simulink model "HydICengine"  (R2023b)
settings: Solver=ode3  StartTime=0.0  StopTime=1*sim_time  FixedStep=(120/engine_speed)/2000  RelTol=1e-3  EnableMultiTasking=on
values from neighbouring files (symbols this model uses):
  engine_speed = 1500    [RunModel.m]
  sim_time = stepsize * (2*1000 - 1)    (= 0.07996)    [RunModel.m]
settings Model: Creator=htsauto  LastModifiedBy=sami
settings SolverCC: AlgebraicLoopSolver=TrustRegion
settings DataIOCC: LimitDataPoints=on  SaveFormat=Array  SignalLoggingSaveFormat=ModelDataLogs  ReturnWorkspaceOutputs=off
settings OptimizationCC: ExpressionDepthLimit=2147483647  LifeSpan=inf
settings DebuggingCC: UnderspecifiedInitializationDetection=Classic  MergeDetectMultiDrivingBlocksExec=none  SolverPrmCheckMsg=warning  FcnCallInpInsideContextMsg=warning  UnconnectedInputMsg=warning  UnconnectedOutputMsg=warning  UnconnectedLineMsg=warning  StateNameClashWarn=warning  SFUnexpectedBacktrackingDiag=warning  SFNoUnconditionalDefaultTransitionDiag=warning  ArithmeticOperatorsInVariantConditions=warning
settings HardwareCC: ProdBitPerPointer=32  ProdBitPerSizeT=32  ProdBitPerPtrDiffT=32  ProdLargestAtomicFloat=None  ProdIntDivRoundTo=Undefined  ProdEndianess=Unspecified  ProdWordSize=32  ProdHWDeviceType=32-bit Generic
settings ModelReferenceCC: EnableRefExpFcnMdlSchedulingChecks=on  PropagateSignalLabelsOutOfModel=off
settings SFSimCC: SimUseLocalCustomCode=off  CustomCodeUndefinedFunction=UseInterfaceOnly
settings RTWCC: RTWUseLocalCustomCode=off
settings CodeAppCC: StateflowObjectComments=on
settings GRTTargetCC: TargetLangStandard=C89/C90 (ANSI)  CombineOutputUpdateFcns=off  GRTInterface=on
settings ConfigComp: CovMetricSettings=dw  CovSaveCumulativeToWorkspaceVar=on  CovSaveSingleToWorkspaceVar=on  CovExternalEMLEnable=off  CovSFcnEnable=off

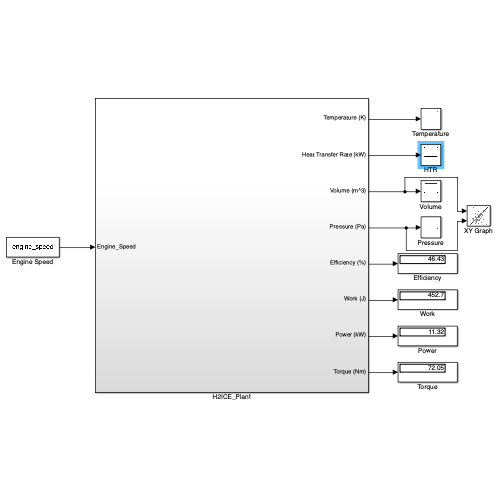
[thumbnail: Simulink's stored preview of the top-level diagram]
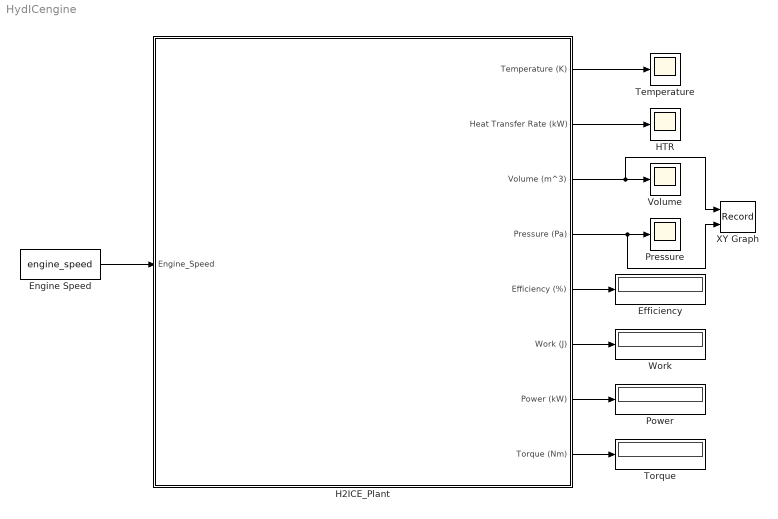
== system HydICengine ==
  Efficiency : Display
  Engine Speed : Constant  Value=engine_speed
  H2ICE_Plant : Subsystem
  HTR : Scope
  Power : Display
  Pressure : Scope
  Temperature : Scope
  Torque : Display
  Volume : Scope
  Work : Display
  XY Graph : Record  FileSettingsInternal="{\"entries\":[{\"content\":{\"excelSettings\":{\"content\":{},\"type\":\"Streamout.ExcelSettings\"}},\"type\":\"Streamout.FileSettingStorage\",\"uuid\":\"\"}],\"packageUris\":[\"http:\\/\\/schema.mathworks.com\\/mf0\\/streamout_blocks\\/R2020a\"],\"version\":\"1.0\"}"  Layout=[1 1]  SignalsInternal="{\"entries\":[{\"content\":{\"signals\":[{\"content\":{\"blockPath\":[],\"dimensions\":[1],\"domain\":\"\",\"lineColor\":\"#fe330a\",\"plots\":[ 1 ],\"port\":1,\"sid\":[\"\"],\"signalID\":1,\"signalName\":\"H2ICE_Plant:3\"},\"type\":\"RecordBlkView.Signal\",\"uuid\":\"\"},{\"content\":{\"blockPath\":[],\"dimensions\":[1],\"domain\":\"\",\"lineColor\":\"#fe330a\",\"plots\":[ 1 ],\"port\":2,\"sid\":[\"\"],\"signalID\":2,\"signalName\":\"H2ICE_Plant:4\"},\"type\":\"RecordBlkView.Signal\",\"uuid\":\"\"}]},\"type\":\"RecordBlkView.InputSignals\",\"uuid\":\"\"}],\"packageUris\":[\"http:\\/\\/schema.mathworks.com\\/mf0\\/streamout_blocks\\/R2020a\"],\"version\":\"1.0\"}"  VisualizationBindings="{\"xyplotplugin\":{\"info\":[{\"series\":[{\"bindingParametersList\":[{\"parameter\":\"X-Axis\",\"signalID\":1,\"signalName\":\"H2ICE_Plant:3\"},{\"parameter\":\"Y-Axis\",\"signalID\":2,\"signalName\":\"H2ICE_Plant:4\"}],\"seriesID\":0}],\"subplotID\":1}]}}"  CompatibilityTag=XY
  wires:
  H2ICE_Plant/8(Torque (Nm)) -> Torque/1
  H2ICE_Plant/7(Power (kW)) -> Power/1
  H2ICE_Plant/6(Work (J)) -> Work/1
  H2ICE_Plant/5(Efficiency (%)) -> Efficiency/1
  H2ICE_Plant/3(Volume (m^3)) -> Volume/1, XY Graph/1
  H2ICE_Plant/4(Pressure (Pa)) -> Pressure/1, XY Graph/2
  H2ICE_Plant/1(Temperature (K)) -> Temperature/1
  Engine Speed/1 -> H2ICE_Plant/1(Engine_Speed)
  H2ICE_Plant/2(Heat Transfer Rate (kW)) -> HTR/1

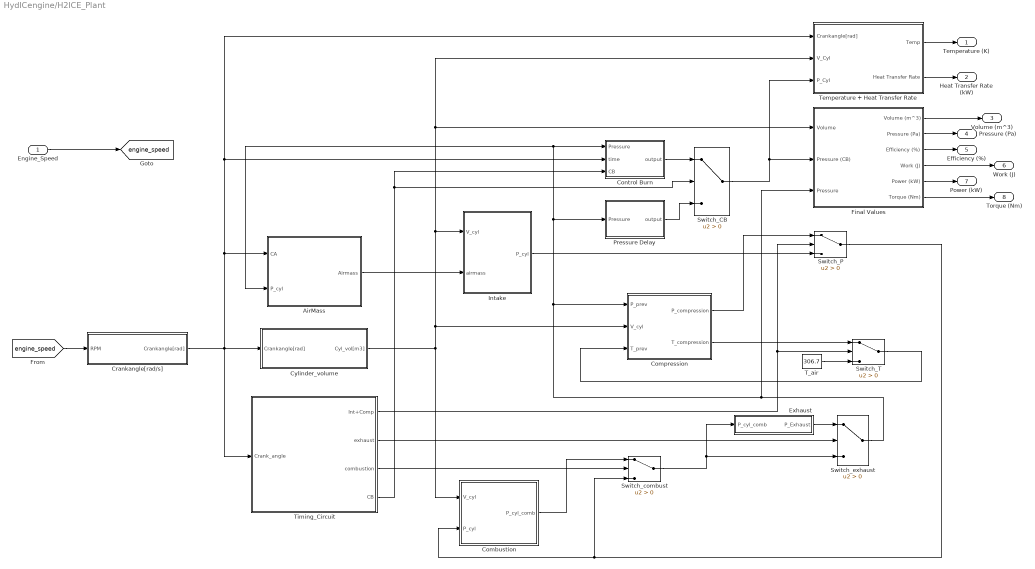
== system HydICengine/H2ICE_Plant ==
  Engine_Speed : Inport
  AirMass : Subsystem
  Combustion : Subsystem
  Compression : Subsystem
  Control Burn : Subsystem
  Crankangle[rad/s] : Subsystem
  Cylinder_volume : Subsystem
  Exhaust : Subsystem
  Final Values : Subsystem
  Intake : Subsystem
  Pressure Delay : Subsystem
  Switch_CB : Switch  Criteria=u2 > Threshold  SaturateOnIntegerOverflow=off  InputSameDT=off
  Switch_P : Switch  Criteria=u2 > Threshold  SaturateOnIntegerOverflow=off  InputSameDT=off
  Switch_T : Switch  Criteria=u2 > Threshold  SaturateOnIntegerOverflow=off  InputSameDT=off
  Switch_combust : Switch  Criteria=u2 > Threshold  SaturateOnIntegerOverflow=off  InputSameDT=off
  Switch_exhaust : Switch  Criteria=u2 > Threshold  SaturateOnIntegerOverflow=off  InputSameDT=off
  T_air : Constant  Value=306.7
  Temperature + Heat Transfer Rate : Subsystem
  Timing_Circuit : Subsystem
  Temperature (K) : Outport
  Heat Transfer Rate (kW) : Outport  Port=2
  Volume (m^3) : Outport  Port=3
  Pressure (Pa) : Outport  Port=4
  Efficiency (%) : Outport  Port=5
  Work (J) : Outport  Port=6
  Power (kW) : Outport  Port=7
  Torque (Nm) : Outport  Port=8
  tag scope: engine_speed=global
  wires:
  [engine_speed] -> Crankangle[rad/s]/1(RPM)
  Switch_exhaust/1 -> Final Values/3(Pressure), AirMass/2(P_cyl), Control Burn/1(Pressure), Pressure Delay/1(Pressure), Compression/1(P_prev)
  Combustion/1(P_cyl_comb) -> Switch_combust/1
  Switch_T/1 -> Compression/3(T_prev)
  Switch_combust/1 -> Exhaust/1(P_cyl_comb), Switch_exhaust/3
  Compression/2(T_compression) -> Switch_T/1
  AirMass/1(Airmass) -> Intake/2(airmass)
  Cylinder_volume/1(Cyl_vol[m3]) -> Compression/2(V_cyl), Temperature + Heat Transfer Rate/2(V_Cyl), Final Values/1(Volume), Intake/1(V_cyl), Combustion/1(V_cyl)
  Exhaust/1(P_Exhaust) -> Switch_exhaust/1
  Compression/1(P_compression) -> Switch_P/1
  Crankangle[rad/s]/1(Crankangle[rad]) -> Timing_Circuit/1(Crank_angle), Temperature + Heat Transfer Rate/1(Crankangle[rad]), Control Burn/2(time), AirMass/1(CA), Cylinder_volume/1(Crankangle[rad])
  T_air/1 -> Switch_T/3
  Intake/1(P_cyl) -> Switch_P/3
  Timing_Circuit/3(combustion) -> Switch_combust/2
  Switch_P/1 -> Combustion/2(P_cyl), Switch_combust/3
  Timing_Circuit/2(exhaust) -> Switch_exhaust/2
  Timing_Circuit/1(Int+Comp) -> Switch_P/2, Switch_T/2
  Temperature + Heat Transfer Rate/2(Heat Transfer Rate) -> Heat Transfer Rate (kW)/1
  Temperature + Heat Transfer Rate/1(Temp) -> Temperature (K)/1
  Final Values/2(Pressure (Pa)) -> Pressure (Pa)/1
  Final Values/1(Volume (m^3)) -> Volume (m^3)/1
  Engine_Speed/1 -> [engine_speed]
  Final Values/3(Efficiency (%)) -> Efficiency (%)/1
  Final Values/4(Work (J)) -> Work (J)/1
  Final Values/5(Power (kW)) -> Power (kW)/1
  Final Values/6(Torque (Nm)) -> Torque (Nm)/1
  Switch_CB/1 -> Temperature + Heat Transfer Rate/3(P_Cyl), Final Values/2(Pressure (CB))
  Timing_Circuit/4(CB) -> Control Burn/3(CB), Switch_CB/2
  Control Burn/1(output) -> Switch_CB/1
  Pressure Delay/1(output) -> Switch_CB/3

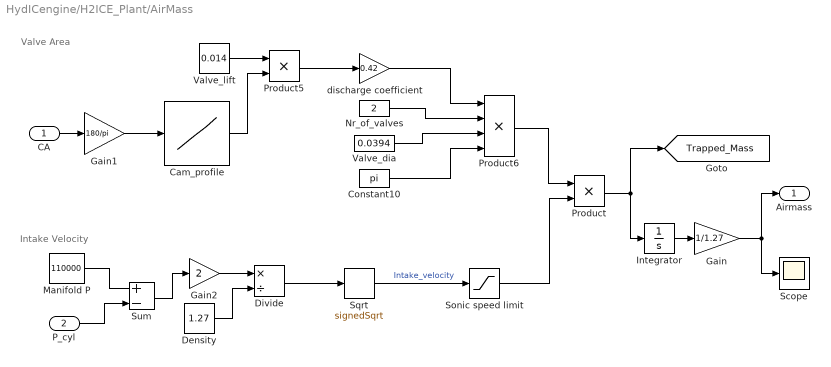
== system HydICengine/H2ICE_Plant/AirMass ==
  note: Intake Velocity
  note: Valve Area
  CA : Inport
  P_cyl : Inport  Port=2
  Cam_profile : Lookup_n-D  NumberOfTableDimensions=1  BreakpointsForDimension1=[0,10,20,30,40,50,60,70,80,90,100,110,120,130,140,150,160,170,180,190,200,210]  Table=[0,0.05,0.1,0.2,0.3,0.5,0.65,0.8,0.9,0.95,1,1,1,1,0.9,0.8,0.65,0.5,0.3,0.2,0.1,0]  ExtrapMethod=Clip  UseLastTableValue=on  RndMeth=Simplest
  Constant10 : Constant  Value=pi
  Density : Constant  Value=1.27
  Divide : Product  Inputs=*/
  Gain : Gain  Gain=1/1.27
  Gain1 : Gain  Gain=180/pi
  Gain2 : Gain  Gain=2
  Integrator : Integrator
  Manifold P : Constant  Value=110000
  Nr_of_valves : Constant  Value=2
  Product : Product
  Product5 : Product  RndMeth=Zero
  Product6 : Product  Inputs=4  RndMeth=Zero
  Scope : Scope
  Sonic speed limit : Saturate  UpperLimit=343.439  LowerLimit=-343.439
  Sqrt : Sqrt  Operator=signedSqrt
  Sum : Sum  Inputs=+-
  Valve_dia : Constant  Value=0.0394
  Valve_lift : Constant  Value=0.014
  discharge coefficient : Gain  Gain=0.42
  Airmass : Outport
  tag scope: Trapped_Mass=global
  wires:
  Gain/1 -> Scope/1, Airmass/1
  Product/1 -> [Trapped_Mass], Integrator/1
  Constant10/1 -> Product6/4
  Valve_dia/1 -> Product6/3
  Nr_of_valves/1 -> Product6/2
  discharge coefficient/1 -> Product6/1
  Sonic speed limit/1 -> Product/2
  Divide/1 -> Sqrt/1
  Sqrt/1 -> Sonic speed limit/1  "Intake_velocity"
  Product5/1 -> discharge coefficient/1
  Cam_profile/1 -> Product5/2
  Product6/1 -> Product/1
  Gain2/1 -> Divide/1
  Valve_lift/1 -> Product5/1
  Gain1/1 -> Cam_profile/1
  Sum/1 -> Gain2/1
  Density/1 -> Divide/2
  Integrator/1 -> Gain/1
  CA/1 -> Gain1/1
  P_cyl/1 -> Sum/2
  Manifold P/1 -> Sum/1

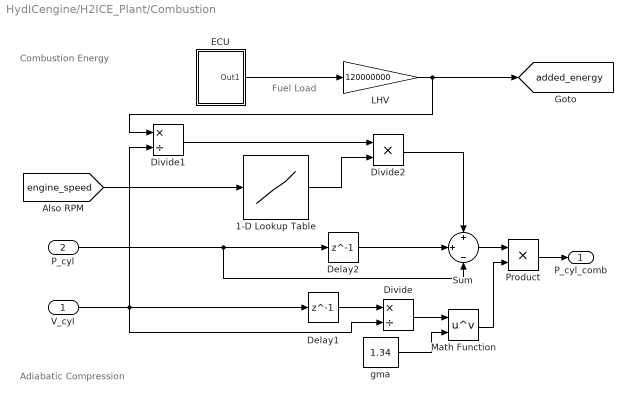
== system HydICengine/H2ICE_Plant/Combustion ==
  note: Combustion Energy
  note: Fuel Load
  note: Adiabatic Compression
  V_cyl : Inport
  P_cyl : Inport  Port=2
  1-D Lookup Table : Lookup_n-D  NumberOfTableDimensions=1  BreakpointsForDimension1=[1000, 1500, 1801, 2000, 2500, 3000, 3500, 4000, 4500, 5000]  Table=[0.36, 0.28, 0.25, 0.23, 0.21, 0.19, 0.19, 0.19, 0.19, 0.19]  InternalRulePriority=Speed  RndMeth=Simplest
  Delay1 : Delay  DelayLength=1
  Delay2 : Delay  DelayLength=1
  Divide : Product  Inputs=*/
  Divide1 : Product  Inputs=*/
  Divide2 : Product  Inputs=**
  ECU : Subsystem
      mask Display: image('Screenshot 2025-03-29 at 14.23.46.png');
  LHV : Gain  Gain=120000000
  Math Function : Math  Operator=pow  SignedPower=on
  Product : Product
  Sum : Sum  Inputs=+|+|-
  gma : Constant  Value=1.34
  P_cyl_comb : Outport
  tag scope: added_energy=global
  wires:
  Delay1/1 -> Divide/1
  Divide/1 -> Math Function/1
  Product/1 -> P_cyl_comb/1
  V_cyl/1 -> Delay1/1, Divide/2, Divide1/2
  Sum/1 -> Product/1
  Delay2/1 -> Sum/2
  Math Function/1 -> Product/2
  gma/1 -> Math Function/2
  P_cyl/1 -> Delay2/1, Sum/3
  [engine_speed] -> 1-D Lookup Table/1
  Divide1/1 -> Divide2/1
  Divide2/1 -> Sum/1
  1-D Lookup Table/1 -> Divide2/2
  LHV/1 -> [added_energy], Divide1/1
  ECU/1(Out1) -> LHV/1

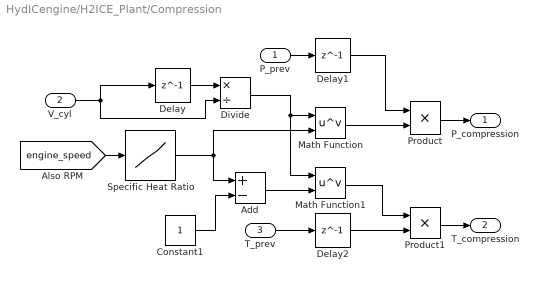
== system HydICengine/H2ICE_Plant/Compression ==
  P_prev : Inport
  V_cyl : Inport  Port=2
  T_prev : Inport  Port=3
  Add : Sum  Inputs=+-
  Constant1 : Constant
  Delay : Delay  DelayLength=1  InitialCondition=0
  Delay1 : Delay  DelayLength=1  InitialCondition=0
  Delay2 : Delay  DelayLength=1
  Divide : Product  Inputs=*/
  Math Function : Math  Operator=pow  SignedPower=on
  Math Function1 : Math  Operator=pow  SignedPower=on
  Product : Product
  Product1 : Product
  Specific Heat Ratio : Lookup_n-D  NumberOfTableDimensions=1  BreakpointsForDimension1=[1000, 1500, 1801, 2000, 2500, 3000, 3500, 4000, 4500, 5000]  Table=[1.6, 1.53, 1.47, 1.45, 1.41, 1.39, 1.38, 1.38, 1.38, 1.38]  InternalRulePriority=Speed  RndMeth=Simplest
  P_compression : Outport
  T_compression : Outport  Port=2
  wires:
  Product1/1 -> T_compression/1
  Delay2/1 -> Product1/2
  Delay1/1 -> Product/1
  Add/1 -> Math Function1/2
  Product/1 -> P_compression/1
  Divide/1 -> Math Function/1, Math Function1/1
  P_prev/1 -> Delay1/1
  Constant1/1 -> Add/2
  V_cyl/1 -> Delay/1, Divide/2
  Math Function/1 -> Product/2
  Math Function1/1 -> Product1/1
  Specific Heat Ratio/1 -> Math Function/2, Add/1
  Delay/1 -> Divide/1
  [engine_speed] -> Specific Heat Ratio/1
  T_prev/1 -> Delay2/1

== system HydICengine/H2ICE_Plant/Control Burn ==
  Pressure : Inport
  time : Inport  Port=2
  CB : Inport  Port=3
  Constant : Constant  Value=6.317760114
  Constant1 : Constant  Value=6.311473785
  Display : Display
  Display1 : Display
  MATLAB Function : MATLAB Function  TreatAsAtomicUnit=on
  MATLAB Function1 : MATLAB Function  TreatAsAtomicUnit=on
  MATLAB Function2 : MATLAB Function  TreatAsAtomicUnit=on
  Scope1 : Scope
  Scope3 : Scope
  output : Outport
  wires:
  Pressure/1 -> MATLAB Function/2(input), MATLAB Function2/1(input)
  Constant/1 -> MATLAB Function/1(targetTime)
  time/1 -> MATLAB Function/3(time), MATLAB Function2/2(time)
  Constant1/1 -> MATLAB Function2/3(targetTime)
  MATLAB Function2/1(output) -> MATLAB Function1/3(minPressure), Display1/1
  MATLAB Function2/2(trigger) -> Scope3/1
  MATLAB Function/1(output) -> MATLAB Function1/1(maxPressure), Display/1
  MATLAB Function1/1(output) -> output/1
  CB/1 -> MATLAB Function1/2(rangeActive)
  MATLAB Function/2(trigger) -> Scope1/1

== system HydICengine/H2ICE_Plant/Crankangle[rad//s] ==
  RPM : Inport
  Clock : Clock
  Display : Display
  Product : Product
  RPM to rad : Gain  Gain=(2*pi/60)
  Scope : Scope
  Crankangle[rad] : Outport
  wires:
  RPM/1 -> RPM to rad/1
  RPM to rad/1 -> Product/1
  Clock/1 -> Product/2
  Product/1 -> Display/1, Scope/1, Crankangle[rad]/1

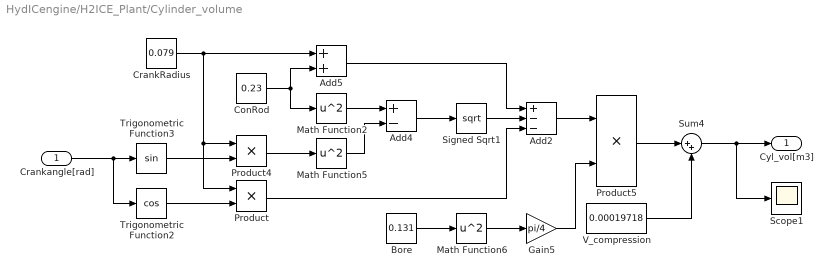
== system HydICengine/H2ICE_Plant/Cylinder_volume ==
  Crankangle[rad] : Inport
  Add2 : Sum  Inputs=+--
  Add4 : Sum  Inputs=+-
  Add5 : Sum
  Bore : Constant  Value=0.131
  ConRod : Constant  Value=0.23
  CrankRadius : Constant  Value=0.079
  Gain5 : Gain  Gain=pi/4
  Math Function2 : Math  Operator=square  SignedPower=on
  Math Function5 : Math  Operator=square  SignedPower=on
  Math Function6 : Math  Operator=square  SignedPower=on
  Product : Product
  Product4 : Product
  Product5 : Product
  Scope1 : Scope
  Signed Sqrt1 : Sqrt
  Sum4 : Sum  Inputs=|++
  Trigonometric Function2 : Trigonometry  Operator=cos
  Trigonometric Function3 : Trigonometry
  V_compression : Constant  Value=0.00019718
  Cyl_vol[m3] : Outport
  wires:
  Product5/1 -> Sum4/1
  Sum4/1 -> Scope1/1, Cyl_vol[m3]/1
  Gain5/1 -> Product5/2
  Add2/1 -> Product5/1
  Math Function6/1 -> Gain5/1
  ConRod/1 -> Add5/2, Math Function2/1
  Add4/1 -> Signed Sqrt1/1
  Product4/1 -> Math Function5/1
  Math Function2/1 -> Add4/1
  V_compression/1 -> Sum4/2
  Add5/1 -> Add2/1
  Product/1 -> Add2/3
  Signed Sqrt1/1 -> Add2/2
  Math Function5/1 -> Add4/2
  Trigonometric Function2/1 -> Product/2
  Crankangle[rad]/1 -> Trigonometric Function2/1, Trigonometric Function3/1
  CrankRadius/1 -> Add5/1, Product4/1, Product/1
  Bore/1 -> Math Function6/1
  Trigonometric Function3/1 -> Product4/2

== system HydICengine/H2ICE_Plant/Exhaust ==
  P_cyl_comb : Inport
  Clock : Clock
  Constant : Constant  Value=sim_time
  Gain : Gain  Gain=0.74
  Relational Operator : RelationalOperator  OutDataTypeStr=boolean  RndMeth=Simplest  InputSameDT=off
  Triggered Subsystem : Subsystem  TreatAsAtomicUnit=on
  P_Exhaust : Outport
  wires:
  Constant/1 -> Gain/1
  Clock/1 -> Relational Operator/1
  Gain/1 -> Relational Operator/2
  Relational Operator/1 -> Triggered Subsystem/Trigger
  P_cyl_comb/1 -> Triggered Subsystem/1(In1)
  Triggered Subsystem/1(Out1) -> P_Exhaust/1

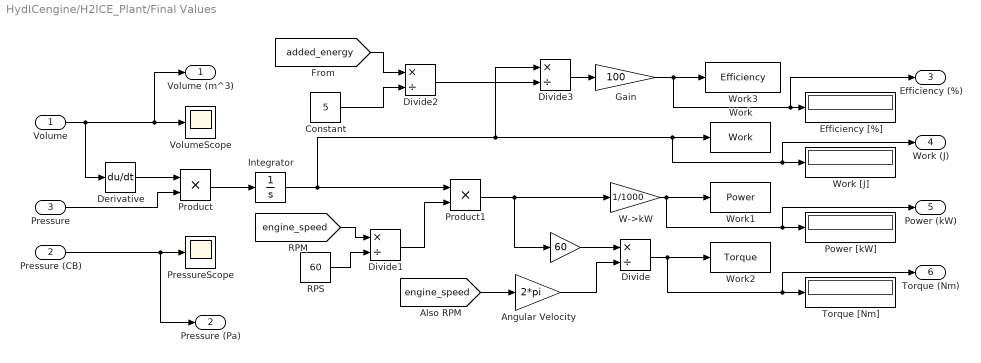
== system HydICengine/H2ICE_Plant/Final Values ==
  Volume : Inport
  Pressure (CB) : Inport  Port=2
  Pressure : Inport  Port=3
  "      " : Gain  Gain=60
  "      W->kW" : Gain  Gain=1/1000
  Angular Velocity : Gain  Gain=2*pi
  Constant : Constant  Value=5
  Derivative : Derivative
  Divide{,1..3} (4 alike) : Product  Inputs=*/
  Efficiency [%] : Display
  Gain : Gain  Gain=100
  Integrator : Integrator
  Power [kW] : Display
  PressureScope : Scope
  Product : Product
  Product1 : Product
  RPS : Constant  Value=60
  Torque [Nm] : Display
  VolumeScope : Scope
  Work : ToWorkspace  VariableName=Work  SampleTime=-1
      settings: MaxDataPoints=1
  "Work [J] " : Display
  Work1 : ToWorkspace  VariableName=Power  SampleTime=-1
      settings: MaxDataPoints=1
  Work2 : ToWorkspace  VariableName=Torque  SampleTime=-1
      settings: MaxDataPoints=1
  Work3 : ToWorkspace  VariableName=Efficiency  SampleTime=-1
      settings: MaxDataPoints=1
  Volume (m^3) : Outport
  Pressure (Pa) : Outport  Port=2
  Efficiency (%) : Outport  Port=3
  Work (J) : Outport  Port=4
  Power (kW) : Outport  Port=5
  Torque (Nm) : Outport  Port=6
  wires:
  Integrator/1 -> Work/1, Work (J)/1, "Work [J] "/1, Divide3/1, Product1/1
  Volume/1 -> Derivative/1, Volume (m^3)/1, VolumeScope/1
  Derivative/1 -> Product/1
  Product/1 -> Integrator/1
  "      "/1 -> Divide/1
  [engine_speed] -> Angular Velocity/1
  Angular Velocity/1 -> Divide/2
  [engine_speed] -> Divide1/1
  RPS/1 -> Divide1/2
  Divide1/1 -> Product1/2
  "      W->kW"/1 -> Power (kW)/1, Power [kW]/1, Work1/1
  [added_energy] -> Divide2/1
  Constant/1 -> Divide2/2
  Divide2/1 -> Divide3/2
  Divide3/1 -> Gain/1
  Gain/1 -> Work3/1, Efficiency (%)/1, Efficiency [%]/1
  Pressure (CB)/1 -> Pressure (Pa)/1, PressureScope/1
  Divide/1 -> Work2/1, Torque (Nm)/1, Torque [Nm]/1
  Pressure/1 -> Product/2
  Product1/1 -> "      W->kW"/1, "      "/1

== system HydICengine/H2ICE_Plant/Intake ==
  note: pre-combustion cylinder pressure
  V_cyl : Inport
  airmass : Inport  Port=2
  Display : Display
  Product7 : Product  Inputs=/***  RndMeth=Zero
  R : Constant  Value=287
  Scope : Scope
  Sum6 : Sum  Inputs=|++
  T_air : Constant  Value=306.7
  To Workspace : ToWorkspace  VariableName=AirMass  SampleTime=-1
      settings: MaxDataPoints=1
  m_0 : Constant  Value=0.00022401
  P_cyl : Outport
  wires:
  R/1 -> Product7/3
  T_air/1 -> Product7/4
  Product7/1 -> Display/1, P_cyl/1, Scope/1
  Sum6/1 -> Product7/2
  m_0/1 -> Sum6/1
  airmass/1 -> To Workspace/1, Sum6/2
  V_cyl/1 -> Product7/1

== system HydICengine/H2ICE_Plant/Pressure Delay ==
  Pressure : Inport
  Delay : Delay  DelayLength=24  InitialCondition=0
  Switch : Switch  Criteria=u2 > Threshold  SaturateOnIntegerOverflow=off  InputSameDT=off
  output : Outport
  wires:
  Pressure/1 -> Delay/1, Switch/1
  Delay/1 -> Switch/3
  [CB2] -> Switch/2
  Switch/1 -> output/1

== system HydICengine/H2ICE_Plant/Temperature + Heat Transfer Rate ==
  Crankangle[rad] : Inport
  V_Cyl : Inport  Port=2
  P_Cyl : Inport  Port=3
  Heat Transfer Rate Subsystem : Subsystem
  Heat_Transfer_Rate : Scope
  Temp Subsystem : Subsystem
  Temperature : Scope
  To Workspace : ToWorkspace  VariableName=Heat_Transfer_Rate  SampleTime=-1
      settings: Save2DSignal=2-D array (concatenate along first dimension)
  Temp : Outport
  Heat Transfer Rate : Outport  Port=2
  wires:
  P_Cyl/1 -> Heat Transfer Rate Subsystem/1(P_Cyl), Temp Subsystem/1(P_Cyl)
  Temp Subsystem/1(Temperature) -> Heat Transfer Rate Subsystem/2(Temperature), Temp/1, Temperature/1
  V_Cyl/1 -> Temp Subsystem/2(V_Cyl)
  Crankangle[rad]/1 -> Temp Subsystem/3(Crankangle[rad]), Heat Transfer Rate Subsystem/3(Crankangle[rad])
  Heat Transfer Rate Subsystem/1(Heat Transfer Rate) -> To Workspace/1, Heat_Transfer_Rate/1, Heat Transfer Rate/1

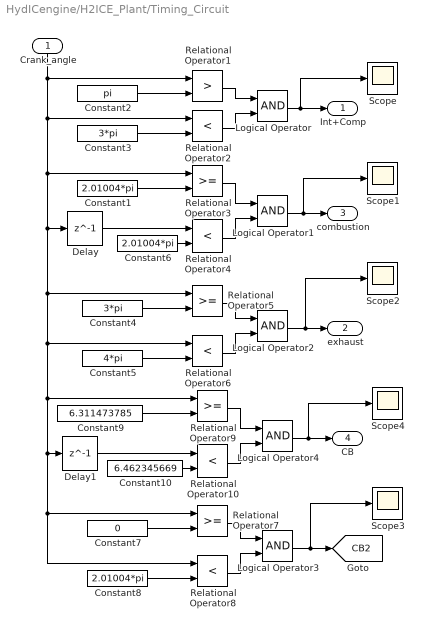
== system HydICengine/H2ICE_Plant/Timing_Circuit ==
  Crank_angle : Inport
  Constant1 : Constant  Value=2.01004*pi
  Constant10 : Constant  Value=6.462345669
  Constant2 : Constant  Value=pi
  Constant3 : Constant  Value=3*pi
  Constant4 : Constant  Value=3*pi
  Constant5 : Constant  Value=4*pi
  Constant6 : Constant  Value=2.01004*pi
  Constant7 : Constant  Value=0
  Constant8 : Constant  Value=2.01004*pi
  Constant9 : Constant  Value=6.311473785
  Delay : Delay  DelayLength=1  InitialCondition=100000
  Delay1 : Delay  DelayLength=1  InitialCondition=100000
  Logical Operator{,1..4} (5 alike) : Logic  AllPortsSameDT=off  OutDataTypeStr=boolean
  Relational Operator1 : RelationalOperator  Operator=>  OutDataTypeStr=boolean  InputSameDT=off
  Relational Operator{2,4,6,8,10} (5 alike) : RelationalOperator  Operator=<  OutDataTypeStr=boolean  InputSameDT=off
  Relational Operator{3,5,7,9} (4 alike) : RelationalOperator  OutDataTypeStr=boolean  InputSameDT=off
  Scope{,1..4} (5 alike) : Scope
  Int+Comp : Outport
  exhaust : Outport  Port=2
  combustion : Outport  Port=3
  CB : Outport  Port=4
  tag scope: CB2=global
  wires:
  Relational Operator6/1 -> Logical Operator2/2
  Logical Operator2/1 -> Scope2/1, exhaust/1
  Relational Operator5/1 -> Logical Operator2/1
  Constant4/1 -> Relational Operator5/2
  Logical Operator/1 -> Scope/1, Int+Comp/1
  Relational Operator3/1 -> Logical Operator1/1
  Relational Operator4/1 -> Logical Operator1/2
  Logical Operator1/1 -> Scope1/1, combustion/1
  Constant2/1 -> Relational Operator1/2
  Constant1/1 -> Relational Operator3/2
  Relational Operator2/1 -> Logical Operator/2
  Relational Operator1/1 -> Logical Operator/1
  Constant3/1 -> Relational Operator2/2
  Constant5/1 -> Relational Operator6/2
  Constant6/1 -> Relational Operator4/2
  Delay/1 -> Relational Operator4/1
  Constant9/1 -> Relational Operator9/2
  Delay1/1 -> Relational Operator10/1
  Relational Operator9/1 -> Logical Operator4/1
  Constant10/1 -> Relational Operator10/2
  Relational Operator10/1 -> Logical Operator4/2
  Logical Operator4/1 -> Scope4/1, CB/1
  Relational Operator8/1 -> Logical Operator3/2
  Relational Operator7/1 -> Logical Operator3/1
  Crank_angle/1 -> Relational Operator6/1, Relational Operator9/1, Relational Operator7/1, Relational Operator8/1, Delay1/1, Relational Operator5/1, Delay/1, Relational Operator3/1, Relational Operator2/1, Relational Operator1/1
  Logical Operator3/1 -> [CB2], Scope3/1
  Constant7/1 -> Relational Operator7/2
  Constant8/1 -> Relational Operator8/2

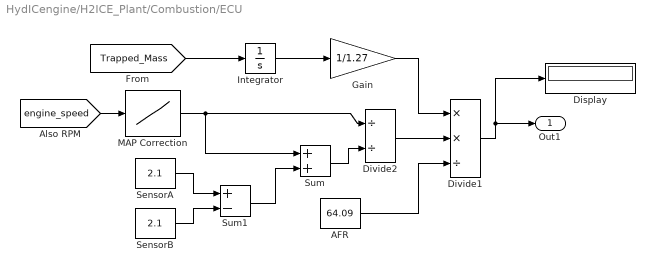
== system HydICengine/H2ICE_Plant/Combustion/ECU ==
  AFR : Constant  Value=64.09
  Display : Display
  Divide1 : Product  Inputs=**/
  Divide2 : Product  Inputs=//
  Gain : Gain  Gain=1/1.27
  Integrator : Integrator
  MAP Correction : Lookup_n-D  NumberOfTableDimensions=1  BreakpointsForDimension1=[1000, 1500, 2000, 2500, 3000, 3500, 4000, 4500, 5000]  Table=[0.9, 1.0, 1.1, 1.2, 1.3, 1.4, 1.5, 1.6, 1.7]  ExtrapMethod=Clip  UseLastTableValue=on  RndMeth=Simplest
  SensorA : Constant  Value=2.1
  SensorB : Constant  Value=2.1
  Sum : Sum
  Sum1 : Sum  Inputs=+-
  Out1 : Outport
  wires:
  Divide1/1 -> Display/1, Out1/1
  [Trapped_Mass] -> Integrator/1
  Gain/1 -> Divide1/1
  Integrator/1 -> Gain/1
  AFR/1 -> Divide1/3
  [engine_speed] -> MAP Correction/1
  MAP Correction/1 -> Sum/1, Divide2/1
  SensorA/1 -> Sum1/1
  SensorB/1 -> Sum1/2
  Sum1/1 -> Sum/2
  Sum/1 -> Divide2/2
  Divide2/1 -> Divide1/2

== system HydICengine/H2ICE_Plant/Exhaust/Triggered Subsystem ==
  In1 : Inport
  Trigger : TriggerPort  VariantControl=(inherit)
  Data Store Memory : DataStoreMemory  DataStoreName=Stored_P_exhaust  WriteAfterWriteMsg=warning  ShowAdditionalParam=off
  Data Store Read : DataStoreRead  DataStoreName=Stored_P_exhaust  IndexOptions=Index vector (dialog)  Indices=1  OutputSizes=1
  Data Store Write : DataStoreWrite  DataStoreName=Stored_P_exhaust  IndexOptions=Index vector (dialog)  Indices=1  OutputSizes=1
  Out1 : Outport
  wires:
  In1/1 -> Data Store Write/1
  Data Store Read/1 -> Out1/1

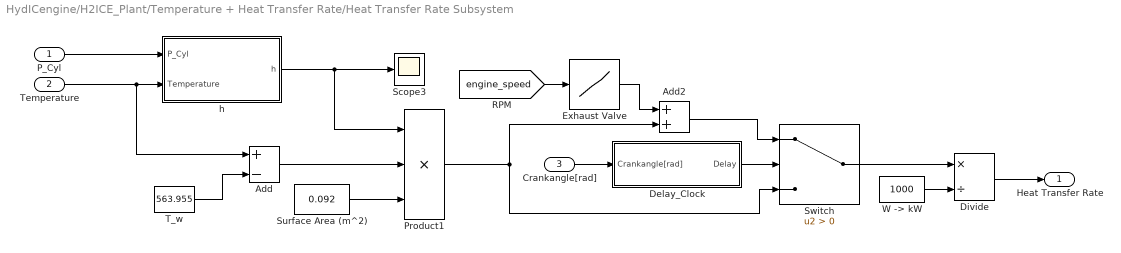
== system HydICengine/H2ICE_Plant/Temperature + Heat Transfer Rate/Heat Transfer Rate Subsystem ==
  P_Cyl : Inport
  Temperature : Inport  Port=2
  Crankangle[rad] : Inport  Port=3
  Add : Sum  Inputs=+-
  Add2 : Sum
  Delay_Clock : Subsystem
  Divide : Product  Inputs=*/
  Exhaust Valve : Lookup_n-D  NumberOfTableDimensions=1  BreakpointsForDimension1=[1000, 1500, 1801, 2000, 2500, 3000, 3500, 4000, 4500, 5000]  Table=[16550.7, 20208.5, 20942.2, 21289.2, 21696.5, 22232.9, 22390.9, 22459.3, 22368.5, 22253.2]  InternalRulePriority=Speed  RndMeth=Simplest
  Product1 : Product  Inputs=3
  Scope3 : Scope
  Surface Area (m^2) : Constant  Value=0.092
  Switch : Switch  Criteria=u2 > Threshold  SaturateOnIntegerOverflow=off  InputSameDT=off
  T_w : Constant  Value=563.955
  "W -> kW" : Constant  Value=1000
  h : Subsystem
  Heat Transfer Rate : Outport
  wires:
  Product1/1 -> Switch/3, Add2/2
  T_w/1 -> Add/2
  Delay_Clock/1(Delay) -> Switch/2
  P_Cyl/1 -> h/1(P_Cyl)
  Temperature/1 -> Add/1, h/2(Temperature)
  h/1(h) -> Scope3/1, Product1/1
  Add/1 -> Product1/2
  Surface Area (m^2)/1 -> Product1/3
  Crankangle[rad]/1 -> Delay_Clock/1(Crankangle[rad])
  Add2/1 -> Switch/1
  Switch/1 -> Divide/1
  Divide/1 -> Heat Transfer Rate/1
  "W -> kW"/1 -> Divide/2
  [engine_speed] -> Exhaust Valve/1
  Exhaust Valve/1 -> Add2/1

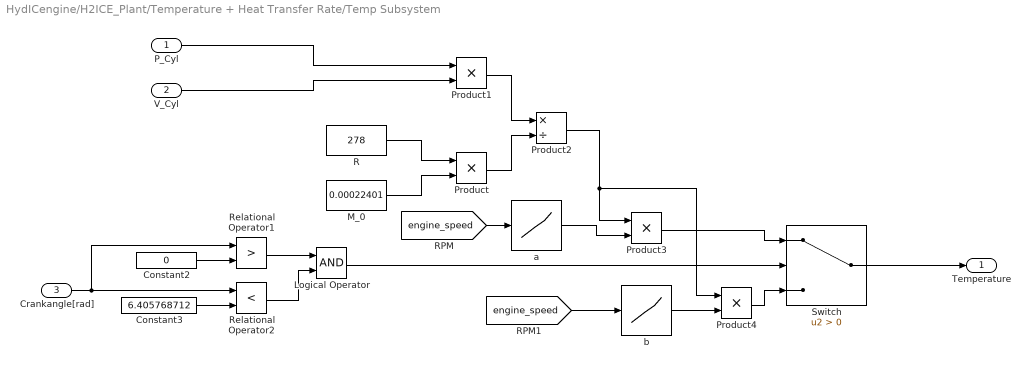
== system HydICengine/H2ICE_Plant/Temperature + Heat Transfer Rate/Temp Subsystem ==
  P_Cyl : Inport
  V_Cyl : Inport  Port=2
  Crankangle[rad] : Inport  Port=3
  Constant2 : Constant  Value=0
  Constant3 : Constant  Value=6.405768712
  Logical Operator : Logic  AllPortsSameDT=off  OutDataTypeStr=boolean
  M_0 : Constant  Value=0.00022401
  Product{,1,3..4} (4 alike) : Product
  Product2 : Product  Inputs=*/
  R : Constant  Value=278
  Relational Operator1 : RelationalOperator  Operator=>  OutDataTypeStr=boolean  InputSameDT=off
  Relational Operator2 : RelationalOperator  Operator=<  OutDataTypeStr=boolean  InputSameDT=off
  Switch : Switch  Criteria=u2 > Threshold  SaturateOnIntegerOverflow=off  InputSameDT=off
  a : Lookup_n-D  NumberOfTableDimensions=1  BreakpointsForDimension1=[1000, 1500, 1801, 2000, 2500, 3000, 3500, 4000, 4500, 5000]  Table=[0.0494, 0.0619, 0.0754, 0.083, 0.1023, 0.1201, 0.1372, 0.1511, 0.1679, 0.1842]  InternalRulePriority=Speed  RndMeth=Simplest
  b : Lookup_n-D  NumberOfTableDimensions=1  BreakpointsForDimension1=[1000, 1500, 1801, 2000, 2500, 3000, 3500, 4000, 4500, 5000]  Table=[0.0636, 0.0831, 0.0961, 0.1079, 0.1293, 0.1567, 0.1713, 0.1866, 0.2017, 0.2147]  InternalRulePriority=Speed  RndMeth=Simplest
  Temperature : Outport
  wires:
  Logical Operator/1 -> Switch/2
  V_Cyl/1 -> Product1/2
  b/1 -> Product4/2
  Product/1 -> Product2/2
  Crankangle[rad]/1 -> Relational Operator2/1, Relational Operator1/1
  Constant2/1 -> Relational Operator1/2
  P_Cyl/1 -> Product1/1
  Relational Operator2/1 -> Logical Operator/2
  a/1 -> Product3/2
  Product1/1 -> Product2/1
  [engine_speed] -> a/1
  [engine_speed] -> b/1
  Constant3/1 -> Relational Operator2/2
  R/1 -> Product/1
  Product2/1 -> Product3/1, Product4/1
  Relational Operator1/1 -> Logical Operator/1
  M_0/1 -> Product/2
  Product3/1 -> Switch/1
  Product4/1 -> Switch/3
  Switch/1 -> Temperature/1

== system HydICengine/H2ICE_Plant/Temperature + Heat Transfer Rate/Heat Transfer Rate Subsystem/Delay_Clock ==
  Crankangle[rad] : Inport
  Constant2 : Constant  Value=3*pi
  Constant3 : Constant  Value=4*pi
  Logical Operator2 : Logic  AllPortsSameDT=off  OutDataTypeStr=boolean
  Relational Operator5 : RelationalOperator  OutDataTypeStr=boolean  InputSameDT=off
  Relational Operator6 : RelationalOperator  Operator=<  OutDataTypeStr=boolean  InputSameDT=off
  Delay : Outport
  wires:
  Relational Operator6/1 -> Logical Operator2/2
  Relational Operator5/1 -> Logical Operator2/1
  Crankangle[rad]/1 -> Relational Operator6/1, Relational Operator5/1
  Constant3/1 -> Relational Operator6/2
  Constant2/1 -> Relational Operator5/2
  Logical Operator2/1 -> Delay/1

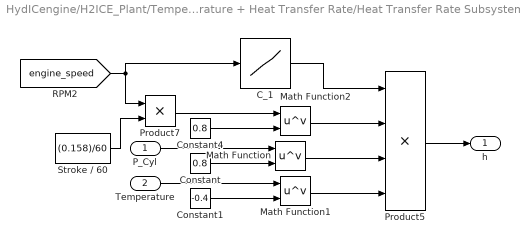
== system HydICengine/H2ICE_Plant/Temperature + Heat Transfer Rate/Heat Transfer Rate Subsystem/h ==
  P_Cyl : Inport
  Temperature : Inport  Port=2
  C_1 : Lookup_n-D  NumberOfTableDimensions=1  BreakpointsForDimension1=[1000, 1500, 1801, 2000, 2500, 3000, 3500, 4000, 4500, 5000]  Table=[0.0486, 0.0391, 0.0384, 0.0338, 0.0300, 0.0286, 0.0260, 0.0243, 0.0231, 0.0225]  InternalRulePriority=Speed  RndMeth=Simplest
  Constant : Constant  Value=0.8
  Constant1 : Constant  Value=-0.4
  Constant4 : Constant  Value=0.8
  Math Function : Math  Operator=pow
  Math Function1 : Math  Operator=pow
  Math Function2 : Math  Operator=pow
  Product5 : Product  Inputs=4
  Product7 : Product
  Stroke / 60 : Constant  Value=(0.158)/60  VectorParams1D=off
  h : Outport
  wires:
  [engine_speed] -> C_1/1, Product7/1
  Stroke / 60/1 -> Product7/2
  Product7/1 -> Math Function2/1
  Math Function/1 -> Product5/3
  P_Cyl/1 -> Math Function/1
  Math Function2/1 -> Product5/2
  Constant/1 -> Math Function/2
  Constant4/1 -> Math Function2/2
  Constant1/1 -> Math Function1/2
  Temperature/1 -> Math Function1/1
  Math Function1/1 -> Product5/4
  Product5/1 -> h/1
  C_1/1 -> Product5/1

== matlab function HydICengine/H2ICE_Plant/Control Burn/MATLAB Function1 ==
  settings: updateMethod=DISCRETE
  data: maxPressure input; rangeActive input; minPressure input; output output
function output = controlledPressureScaling(maxPressure,rangeActive, minPressure)
    persistent activeScaling;
    persistent scaleIndex;
    persistent lastOutput;

    if isempty(activeScaling)
        activeScaling = false;
        scaleIndex = 0;
        lastOutput = minPressure; 
    end

    if rangeActive == 1
        if ~activeScaling
            activeScaling = true;
            scaleIndex = 0;
            lastOutput = minPressure;  
        end
    else
        activeScaling = false;
        lastOutput = 0;
        output = 0;
        return;
    end
    
    if activeScaling
        totalSteps = 25; 
        if scaleIndex < totalSteps - 2
            scale = sin(pi * scaleIndex / totalSteps - pi/2) / 2 + 0.5;
            lastOutput = minPressure + (maxPressure - minPressure) * scale;
            scaleIndex = scaleIndex + 1; 
        elseif scaleIndex >= totalSteps - 2 && scaleIndex <= totalSteps
            lastOutput = maxPressure;
            scaleIndex = scaleIndex + 1; 
            if scaleIndex > totalSteps
                activeScaling = false;  
            end
        end
    end

    output = lastOutput;
end

== matlab function HydICengine/H2ICE_Plant/Control Burn/MATLAB Function ==
  settings: updateMethod=DISCRETE
  data: targetTime input; input input; output output; time input; trigger output
function [output, trigger] = captureComb(targetTime, input, time)
    persistent closestValue;
    persistent minGap;
    
    if isempty(closestValue)
        closestValue = 0; 
        minGap = inf;     
    end

    currentGap = abs(time - targetTime);

    if currentGap < minGap
        closestValue = input; 
        minGap = currentGap;  
        trigger = true;       
    else
        trigger = false;     
    end

    output = closestValue;
end

== matlab function HydICengine/H2ICE_Plant/Control Burn/MATLAB Function2 ==
  settings: updateMethod=DISCRETE
  data: input input; output output; time input; targetTime input; trigger output
function [output, trigger] = captureComp(input, time, targetTime)
    persistent closestValue;
    persistent minGap;
    
    if isempty(closestValue)
        closestValue = 0; 
        minGap = inf;     
    end

    currentGap = abs(time - targetTime);

    if currentGap < minGap
        closestValue = input; 
        minGap = currentGap;  
        trigger = true;       
    else
        trigger = false;   
    end

    output = closestValue;
end
